simulink model "half_car_model_active_suspension"  (R2023b)
settings: Solver=VariableStepAuto  StartTime=0.0  StopTime=20  RelTol=1e-3
values from neighbouring files (symbols this model uses):
  delta0 = -m*g/(2*k)    (= -0.24525)    [half_car_active_suspensions.m]
  Ks = [Ks_controllable, zeros(2,2)]    [half_car_active_suspensions.m]
  p = [ m ... (first row only)    [half_car_active_suspensions.m]
  r0 = 0.1    [half_car_active_suspensions.m]
  u0 = [0;k*delta0*(df-dr)]    [half_car_active_suspensions.m]
  x0 = [  -m*g/(2*k) ... (first row only)    [half_car_active_suspensions.m]
  x0_lin = [ ... (first row only)    [half_car_active_suspensions.m]
libraries: simulink x1
settings Model: Creator=alex2  LastModifiedBy=alex2

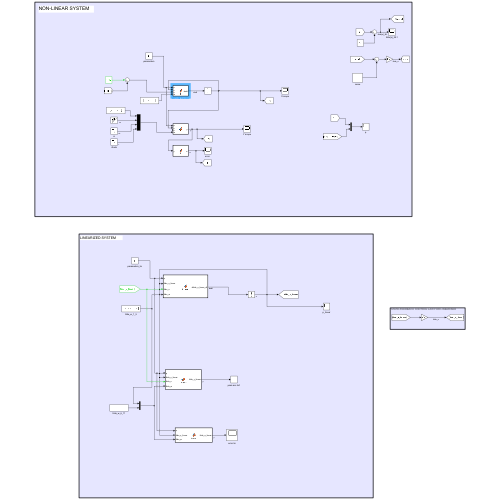
[thumbnail: Simulink's stored preview of the top-level diagram]
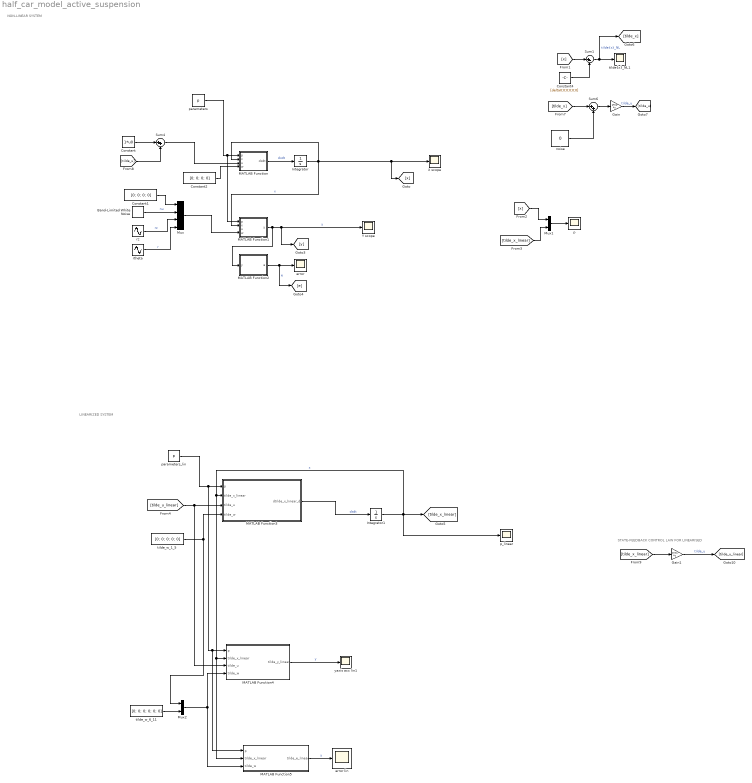
== system half_car_model_active_suspension ==
  note: LINEARIZED SYSTEM
  note: NON-LINEAR SYSTEM
  note: STATE-FEEDBACK CONTROL LAW FOR LINEARISED
  " error lin" : Scope
  Band-Limited White Noise : simulink/Sources/Band-Limited White Noise  Cov="1*[0.00001*1e-2; 0.00001*1e-2;  0.00001*1e-2; 0.00001*1e-2; 0.00001*1e-2]"  Ts=1e-2  seed=[23341; 31826; 11111; 81818; 00001]
  Constant : Constant  Value=1*u0
  Constant1 : Constant  Value=[0; 0; 0; 0]
  Constant2 : Constant  Value=[0; 0; 0; 0]
  Constant4 : Constant  Value=[delta0;0;0;0;0;0]
  Gain : Gain  Gain=1*Ks  Multiplication=Matrix(K*u)
  Gain1 : Gain  Gain=1*Ks  Multiplication=Matrix(K*u)
  Integrator : Integrator  InitialCondition=x0
  Integrator1 : Integrator  InitialCondition=x0_lin
  MATLAB Function : MATLAB Function  TreatAsAtomicUnit=on
  MATLAB Function1 : MATLAB Function  TreatAsAtomicUnit=on
  MATLAB Function2 : MATLAB Function  TreatAsAtomicUnit=on
  MATLAB Function3 : MATLAB Function  TreatAsAtomicUnit=on
  MATLAB Function4 : MATLAB Function  TreatAsAtomicUnit=on
  MATLAB Function5 : MATLAB Function  TreatAsAtomicUnit=on
  Mux : Mux
  Mux1 : Mux  Inputs=2
  Mux2 : Mux  Inputs=2
  Sum1 : Sum  Inputs=|+-
  Sum4 : Sum  Inputs=|++
  Sum6 : Sum  Inputs=|++
  X scope : Scope
  Y scope : Scope
  "error " : Scope
  noise : Constant  Value=0
  p : Scope
  p_linear : Scope
  parameters : Constant  Value=p
  parameters_lin : Constant  Value=p
  rtheta : Sin  Amplitude=0  Bias=r0  Frequency=0  SampleTime=0
  rz : Sin  Amplitude=0  Bias=r0  Frequency=0  SampleTime=0
  tilde_w_1_5 : Constant  Value=[0; 0; 0; 0; 0]
  tilde_w_6_11 : Constant  Value=[0; 0; 0; 0; 0; 0]
  "tilde{x}_NL1" : Scope
  yaxis acc lin1 : Scope
  wires:
  MATLAB Function/1(dxdt) -> Integrator/1  "dxdt"
  Integrator/1 -> MATLAB Function1/2(x), [x], X scope/1, MATLAB Function/2(x)  "x"
  Band-Limited White Noise/1 -> Mux/2  "nu"
  rz/1 -> Mux/3  "rz"
  Constant1/1 -> Mux/1
  Mux/1 -> MATLAB Function1/4(w)
  Constant2/1 -> MATLAB Function/4(w)
  MATLAB Function1/1(y) -> Y scope/1, [y], MATLAB Function2/1(y)  "y"
  rtheta/1 -> Mux/4  "r"
  MATLAB Function2/1(e) -> [e], "error "/1  "e"
  tilde_w_1_5/1 -> Mux2/1, MATLAB Function3/4(tilde_w)
  [tilde_u_linear] -> MATLAB Function4/3(tilde_u), MATLAB Function3/3(tilde_u)
  MATLAB Function3/1(dtilde_x_linear_dt) -> Integrator1/1  "dxdt"
  Integrator1/1 -> p_linear/1, MATLAB Function5/2(tilde_x_linear), MATLAB Function4/2(tilde_x_linear), MATLAB Function3/2(tilde_x_linear), [tilde_x_linear]  "x"
  parameters/1 -> MATLAB Function1/1(p), MATLAB Function/1(p)
  parameters_lin/1 -> MATLAB Function5/1(p), MATLAB Function4/1(p), MATLAB Function3/1(p)
  Mux2/1 -> MATLAB Function4/4(tilde_w), MATLAB Function5/3(tilde_w)
  tilde_w_6_11/1 -> Mux2/2
  MATLAB Function5/1(tilde_e_linear) -> " error lin"/1  "y"
  [tilde_u] -> Sum4/2
  Constant/1 -> Sum4/1
  Sum4/1 -> MATLAB Function/3(u)
  noise/1 -> Sum6/2
  Sum6/1 -> Gain/1
  [tilde_x] -> Sum6/1
  Gain/1 -> [tilde_u]  "tilde_u"
  Sum1/1 -> [tilde_x], "tilde{x}_NL1"/1  "tilde{x}_NL"
  [x] -> Sum1/1
  Constant4/1 -> Sum1/2
  Gain1/1 -> [tilde_u_linear]  "tilde_u"
  [tilde_x_linear] -> Gain1/1
  MATLAB Function4/1(tilde_y_linear) -> yaxis acc lin1/1  "y"
  Mux1/1 -> p/1
  [x] -> Mux1/1
  [tilde_x_linear] -> Mux1/2

== matlab function half_car_model_active_suspension/MATLAB Function1 ==
  data: p input; x input; u input; y output; w input
function y = h(p,x, u, w)

%% parameters
m = p(1);      % [kg] mass
k = p(2);    % [N/m] spring stiffness
beta = p(3);   % [N/(m/s)] damper coeff.
ell0 = p(4);   % [m] 0-load lenght
g = p(5);   % [m/s^2] gravity acceleration
df = p(6);     % [m] distance between center of mass and front
dr = p(7);     % [m] distance between center of mass and rear
J = p(8);      % [kg*m^2] Moment of intertia

%% state
pz = x(1);        % [m] heigth of the center of mass of the car 
vz = x(2);        % [m/s] speed of the center of mass of the car 
ptheta = x(3);    % [Rad] pitch angle of the car 
vtheta = x(4);    % [Rad/s] angular speed of the car 
thetaroad = x(5); % [Rad]Road slope
zroad = x(6);     %[m]Road height 

%% state evolution

s1 = pz+df*(sin(ptheta)-sin(thetaroad)); % height of front suspension
s3 = pz-dr*(sin(ptheta)-sin(thetaroad)); % height of rear suspension

s2 = vz+df*(vtheta*cos(ptheta)-zroad*cos(thetaroad)); % height speed of front suspension
s4 = vz-dr*(vtheta*cos(ptheta)-zroad*cos(thetaroad)); % height speed of rear suspension

lf = s1 + ell0;
lr = s3 + ell0;

%f2 = -g + (((-k*(s1-ell0)-beta*s2)+(-k*(s3-ell0)-beta*s4))+u(1))/m; %  con ell0
%f4 = (df*(-k*(s1-ell0)-beta*s2)-dr*(-k*(s3-ell0)-beta*s4)+u(2)+fwfront*lf+fwrear*lr)/J; %

f2 = -g + (((-k*(s1)-beta*s2)+(-k*(s3)-beta*s4))+u(1))/m; % senza ell0
%f4 = (df*(-k*(s1)-beta*s2)-dr*(-k*(s3)-beta*s4)+u(2)+fwfront*lf+fwrear*lr)/J; %


zgsecond = w(1);
alphag = w(2);
fwfront = w(3);
fwrear = w(4);
nuy = w(5);
nuz = w(6);
nug = w(7);
nuf = w(8);
nur = w(9);

%% reference
rz = w(10);
rtheta=w(11);


%% output
y = [sin(x(3))*(f2 + g) + cos(x(3)) * ((fwrear + fwfront) / m)+nuy; 
     cos(x(3))*(f2 + g) - sin(x(3)) * ((fwrear + fwfront) / m)+nuz; %se facciamo cosi ci da in condizioni stazionarie Zaxisacc=9.81, se vogliamo il valore negativo mettere "-" davanti a coseno 
     x(4)+nug;
     s1+nuf;
     s3+nur;
     rz;
     rtheta];
end

== matlab function half_car_model_active_suspension/MATLAB Function ==
  data: p input; x input; u input; dxdt output; w input
function dxdt = f(p,x,u,w)
%% parameters
%% parameters
m = p(1);      % [kg] mass
k = p(2);    % [N/m] spring stiffness
beta = p(3);   % [N/(m/s)] damper coeff.
ell0 = p(4);   % [m] 0-load lenght
g = p(5);   % [m/s^2] gravity acceleration
df = p(6);     % [m] distance between center of mass and front
dr = p(7);     % [m] distance between center of mass and rear
J = p(8);      % [kg*m^2] Moment of interti
%% state
pz = x(1);        % [m] heigth of the center of mass of the car 
vz = x(2);        % [m/s] speed of the center of mass of the car 
ptheta = x(3);    % [Rad] pitch angle of the car 
vtheta = x(4);    % [Rad/s] angular speed of the car 
thetaroad = x(5); % [Rad]Road slope
zroad = x(6);     %[m]Road height 

%% disturbance
zgsecond = w(1);
alphag = w(2);
fwfront = w(3);
fwrear = w(4);

%todo: Vedere se servono due disturbi 

%% state evolution

s1 = pz+df*(sin(ptheta)-sin(thetaroad)); % height of front suspension
s3 = pz-dr*(sin(ptheta)-sin(thetaroad)); % height of rear suspension

s2 = vz+df*(vtheta*cos(ptheta)-zroad*cos(thetaroad)); % height speed of front suspension
s4 = vz-dr*(vtheta*cos(ptheta)-zroad*cos(thetaroad)); % height speed of rear suspension

lf = s1 + ell0;
lr = s3 + ell0;

%f2 = -g + (((-k*(s1-ell0)-beta*s2)+(-k*(s3-ell0)-beta*s4))+u(1))/m; %  con  ell0
%f4 = (df*(-k*(s1-ell0)-beta*s2)-dr*(-k*(s3-ell0)-beta*s4)+u(2)+fwfront*lf+fwrear*lr)/J; %

f2 = -g + (((-k*(s1)-beta*s2)+(-k*(s3)-beta*s4))+u(1))/m; %  senza ell0
f4 = (df*(-k*(s1)-beta*s2)-dr*(-k*(s3)-beta*s4)+u(2)+fwfront*lf+fwrear*lr)/J; %

dxdt = [vz;
        f2-zgsecond; 
        x(4);
        f4;
        x(6);
        alphag];
        




end

== matlab function half_car_model_active_suspension/MATLAB Function2 ==
  data: y input; e output
function e = E(y)

df = 1;     % [m] distance between center of mass and front
dr = 1;     % [m] distance between center of mass and rear


yy = y(1); % output of h block yaxisacc 
yz = y(2); % output of h block zaxisacc 
yg = y(3); % output of h block gyro
yf = y(4); % output of h block pot. front
yr = y(5); % output of h block pot. rear
 
%% ref
rz = y(6);
rtheta = y(7);

e = [
    (yf*dr+yr*df)/(dr+df)-rz; 
    asin((yy)/(sqrt(yy^2+yz^2)))-rtheta];
end

== matlab function half_car_model_active_suspension/MATLAB Function3 ==
  data: p input; tilde_x_linear input; tilde_u input; dtilde_x_linear_dt output; tilde_w input
function dtilde_x_linear_dt = Linear(p,tilde_x_linear,tilde_u,tilde_w)



%% parameters

%% parameters
m = p(1);      % [kg] mass
k = p(2);    % [N/m] spring stiffness
beta = p(3);   % [N/(m/s)] damper coeff.
ell0 = p(4);   % [m] 0-load lenght
g = p(5);   % [m/s^2] gravity acceleration
df = p(6);     % [m] distance between center of mass and front
dr = p(7);     % [m] distance between center of mass and rear
J = p(8);      % [kg*m^2] Moment of interti


delta0 = -m*g/(2*k);

A = [0, 1, 0, 0, 0, 0;
    -2*k/m, -2*beta/m, -k*(df-dr)/m, -beta*(df-dr)/m, k*(df-dr)/m, beta*(df-dr)/m;
    0, 0, 0, 1, 0, 0;
    -k*(df-dr)/J, -beta*(df-dr)/J, -k*(df^2+dr^2)/J, -beta*(df^2+dr^2)/J, k*(df^2+dr^2)/J, beta*(df^2+dr^2)/J;
    0, 0, 0, 0, 0, 1;
    0, 0, 0, 0, 0, 0];


B1 = [0,0;
     1/m, 0;
     0,0;
     0, 1/J;
     0,0;
     0,0];

B2 = [0,0,0,0,0;
      -1,0,0,0,0;
      0,0,0,0,0;
      0,0,(delta0+ell0)/J,(delta0+ell0)/J, 0;
      0,0,0,0,0;
      0,1,0,0,0];




%% state evolution
dtilde_x_linear_dt = A*tilde_x_linear+B1*tilde_u+B2*tilde_w;
end

== matlab function half_car_model_active_suspension/MATLAB Function4 ==
  data: p input; tilde_x_linear input; tilde_u input; tilde_y_linear output; tilde_w input
function tilde_y_linear = Linear(p,tilde_x_linear,tilde_u,tilde_w)


%% parameters
m = p(1);      % [kg] mass
k = p(2);    % [N/m] spring stiffness
beta = p(3);   % [N/(m/s)] damper coeff.
ell0 = p(4);   % [m] 0-load lenght
g = p(5);   % [m/s^2] gravity acceleration
df = p(6);     % [m] distance between center of mass and front
dr = p(7);     % [m] distance between center of mass and rear
J = p(8);      % [kg*m^2] Moment of interti



C = [0, 0, g, 0, 0, 0;
    -2*k/m, -2*beta/m, -k*(df-dr)/m, -beta*(df-dr)/m, k*(df-dr)/m, beta*(df-dr)/m;
    0, 0, 0, 1, 0, 0;
    1, 0, df, 0, -df, 0;
    1, 0, -dr, 0, dr, 0];


D1 = [0,0;
     1/m, 0;
     0,0;
     0,0;
     0,0];

D2 = [0,0,1/m,1/m,1,0,0,0,0,0,0;
      0,0,0,0,0,1,0,0,0,0,0;
      0,0,0,0,0,0,1,0,0,0,0;
      0,0,0,0,0,0,0,1,0,0,0;
      0,0,0,0,0,0,0,0,1,0,0];




%% state evolution
tilde_y_linear = C*tilde_x_linear+D1*tilde_u+D2*tilde_w;
end

== matlab function half_car_model_active_suspension/MATLAB Function5 ==
  data: p input; tilde_x_linear input; tilde_e_linear output; tilde_w input
function tilde_e_linear = Linear(p,tilde_x_linear,tilde_w)


%% parameters
m = p(1);      % [kg] mass
k = p(2);    % [N/m] spring stiffness
beta = p(3);   % [N/(m/s)] damper coeff.
ell0 = p(4);   % [m] 0-load lenght
g = p(5);   % [m/s^2] gravity acceleration
df = p(6);     % [m] distance between center of mass and front
dr = p(7);     % [m] distance between center of mass and rear
J = p(8);      % [kg*m^2] Moment of interti



Ce = [1,0,0,0,0,0;
      0,0,1,0,0,0];



De2 = [0,0,0,0,0,0,0,dr/(dr+df),df/(dr+df),-1,0;
       0,0, 1/(m*g),1/(m*g),1/g,0,0,0,0,0,-1];




%% state evolution
tilde_e_linear = Ce*tilde_x_linear+De2*tilde_w;
end
